simulink model "boost_rom_lpv_seed7"  (R2026a)
settings: Solver=ode1  StopTime=1.4  FixedStep=5e-07
PreLoadFcn:
  | mdlDir = fileparts(which('boost_rom_lpv_seed7'));
  | repoRoot = fileparts(mdlDir);
  | load(fullfile(repoRoot, 'model_data', 'boost_rom_lpv_seed7_data.mat'));
  | load(fullfile(repoRoot, 'model_data', 'comparison_duty_profile.mat'));
values from neighbouring files (symbols this model uses):
  node_state_ic = [Vout_init; iL_init]    [setup_comparison_profile.m]
undefined symbols (not defined in the file or in its folder): lut_delta_iL, lut_duty, net_lpv, node_u_mean, node_u_std, node_x_mean, node_x_std
libraries: dlconvfclib x3, dlactivationlib x2
settings Model: Creator=arkadiyturevskiy  LastModifiedBy=arkadiyturevskiy

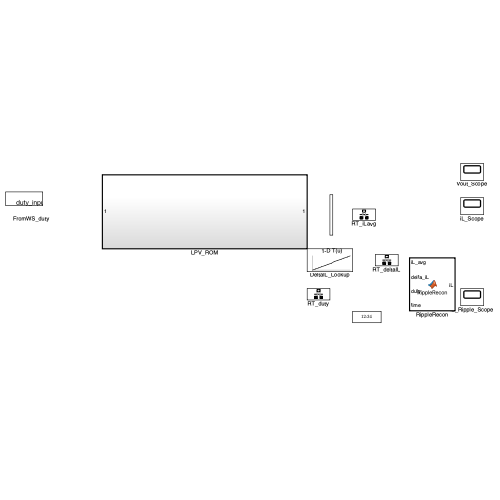
[thumbnail: Simulink's stored preview of the top-level diagram]
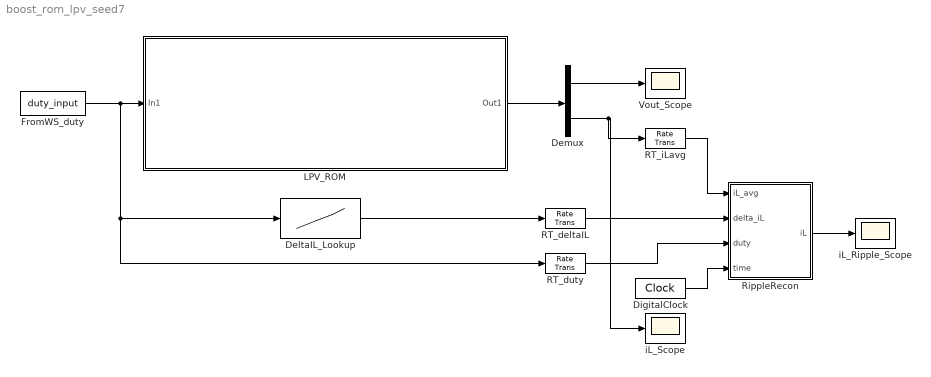
== system boost_rom_lpv_seed7 ==
  DeltaIL_Lookup : Lookup_n-D  NumberOfTableDimensions=1  BreakpointsForDimension1=lut_duty  Table=lut_delta_iL  ExtrapMethod=Clip  InternalRulePriority=Speed  RndMeth=Simplest
  Demux : Demux  Outputs=2
  DigitalClock : DigitalClock  SampleTime=5e-07
  FromWS_duty : FromWorkspace  VariableName=duty_input  OutputAfterFinalValue=Holding final value
  LPV_ROM : Subsystem  TreatAsAtomicUnit=on  SystemSampleTime=5e-06
  RT_deltaIL : RateTransition  OutPortSampleTime=5e-07
  RT_duty : RateTransition  OutPortSampleTime=5e-07
  RT_iLavg : RateTransition  OutPortSampleTime=5e-07
  RippleRecon : MATLAB Function  TreatAsAtomicUnit=on
  Vout_Scope : Scope
  iL_Ripple_Scope : Scope
  iL_Scope : Scope
  wires:
  RippleRecon/1(iL) -> iL_Ripple_Scope/1
  RT_iLavg/1 -> RippleRecon/1(iL_avg)
  RT_duty/1 -> RippleRecon/3(duty)
  RT_deltaIL/1 -> RippleRecon/2(delta_iL)
  Demux/2 -> RT_iLavg/1, iL_Scope/1
  FromWS_duty/1 -> DeltaIL_Lookup/1, RT_duty/1, LPV_ROM/1(In1)
  Demux/1 -> Vout_Scope/1
  DigitalClock/1 -> RippleRecon/4(time)
  DeltaIL_Lookup/1 -> RT_deltaIL/1
  LPV_ROM/1(Out1) -> Demux/1

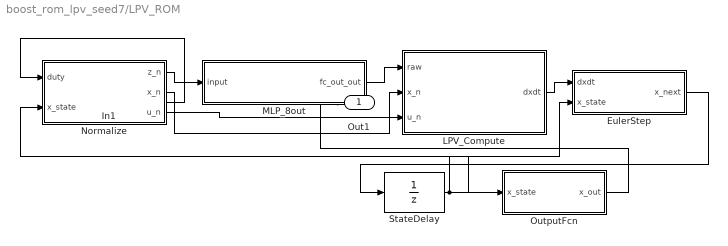
== system boost_rom_lpv_seed7/LPV_ROM ==
  In1 : Inport
  EulerStep : MATLAB Function  TreatAsAtomicUnit=on
  LPV_Compute : MATLAB Function  TreatAsAtomicUnit=on
  MLP_8out : Subsystem
  Normalize : MATLAB Function  TreatAsAtomicUnit=on
  OutputFcn : MATLAB Function  TreatAsAtomicUnit=on
  StateDelay : UnitDelay  InitialCondition=node_state_ic  SampleTime=5e-06
  Out1 : Outport
  wires:
  In1/1 -> Normalize/1(duty)
  StateDelay/1 -> Normalize/2(x_state), EulerStep/2(x_state), OutputFcn/1(x_state)
  Normalize/1(z_n) -> MLP_8out/1(input)
  MLP_8out/1(fc_out_out) -> LPV_Compute/1(raw)
  Normalize/2(x_n) -> LPV_Compute/2(x_n)
  Normalize/3(u_n) -> LPV_Compute/3(u_n)
  LPV_Compute/1(dxdt) -> EulerStep/1(dxdt)
  EulerStep/1(x_next) -> StateDelay/1
  OutputFcn/1(x_out) -> Out1/1

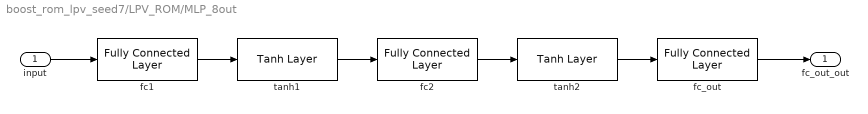
== system boost_rom_lpv_seed7/LPV_ROM/MLP_8out ==
  input : Inport  PortDimensions=[3]  SampleTime=5e-06
  fc1 : dlconvfclib/Fully Connected Layer  Layer=net_lpv.Layers(2)  OutMin=[]  OutMax=[]  WeightsDataTypeStr=Inherit: Inherit via back propagation  WeightsMin=[]  WeightsMax=[]  BiasDataTypeStr=Inherit: Inherit via back propagation  BiasMin=[]  BiasMax=[]  AccumMin=[]  AccumMax=[]  InternalRndMeth=Floor  InternalSaturateOnIntegerOverflow=off  SampleTime=5e-06
      settings: DataFormat=C
  fc2 : dlconvfclib/Fully Connected Layer  Layer=net_lpv.Layers(4)  OutMin=[]  OutMax=[]  WeightsDataTypeStr=Inherit: Inherit via back propagation  WeightsMin=[]  WeightsMax=[]  BiasDataTypeStr=Inherit: Inherit via back propagation  BiasMin=[]  BiasMax=[]  AccumMin=[]  AccumMax=[]  InternalRndMeth=Floor  InternalSaturateOnIntegerOverflow=off  SampleTime=5e-06
      settings: DataFormat=C
  fc_out : dlconvfclib/Fully Connected Layer  Layer=net_lpv.Layers(6)  OutMin=[]  OutMax=[]  WeightsDataTypeStr=Inherit: Inherit via back propagation  WeightsMin=[]  WeightsMax=[]  BiasDataTypeStr=Inherit: Inherit via back propagation  BiasMin=[]  BiasMax=[]  AccumMin=[]  AccumMax=[]  InternalRndMeth=Floor  InternalSaturateOnIntegerOverflow=off  SampleTime=5e-06
      settings: DataFormat=C
  tanh1 : dlactivationlib/Tanh Layer  ApproximationMethod=None  OutMin=[]  OutMax=[]  SampleTime=5e-06
  tanh2 : dlactivationlib/Tanh Layer  ApproximationMethod=None  OutMin=[]  OutMax=[]  SampleTime=5e-06
  fc_out_out : Outport
  wires:
  tanh2/1 -> fc_out/1
  tanh1/1 -> fc2/1
  fc1/1 -> tanh1/1
  input/1 -> fc1/1
  fc_out/1 -> fc_out_out/1
  fc2/1 -> tanh2/1

== matlab function boost_rom_lpv_seed7/LPV_ROM/LPV_Compute ==
  data: raw input; dxdt output; x_n input; u_n input; node_dxdt_scale parameter
function dxdt = LPV_Compute(raw, x_n, u_n, node_dxdt_scale)
%#codegen
% raw: 8-element vector [A(4), B(2), c(2)]
% x_n: 2-element normalized state
% u_n: scalar normalized input
A = reshape(raw(1:4), [2, 2]);
B = reshape(raw(5:6), [2, 1]);
c = raw(7:8);
dxdt_n = A * x_n + B * u_n + c;
dxdt = double(dxdt_n) .* node_dxdt_scale;

== matlab function boost_rom_lpv_seed7/LPV_ROM/Normalize ==
  data: duty input; z_n output; x_state input; x_n output; u_n output; node_x_mean parameter; node_x_std parameter; node_u_mean parameter; node_u_std parameter
function [z_n, x_n, u_n] = Normalize(duty, x_state, node_x_mean, node_x_std, node_u_mean, node_u_std)
%#codegen
x_n = (x_state - node_x_mean) ./ node_x_std;
u_n = (duty - node_u_mean) / node_u_std;
z_n = single([x_n; u_n]);

== matlab function boost_rom_lpv_seed7/LPV_ROM/EulerStep ==
  data: dxdt input; x_next output; x_state input
function x_next = EulerStep(dxdt, x_state)
%#codegen
Ts = 5.0000000000e-06;
x_next = x_state + Ts * dxdt;

== matlab function boost_rom_lpv_seed7/LPV_ROM/OutputFcn ==
  data: x_state input; x_out output
function x_out = OutputFcn(x_state)
%#codegen
x_out = x_state;

== matlab function boost_rom_lpv_seed7/RippleRecon ==
  data: iL_avg input; iL output; delta_iL input; duty input; time input
function iL = RippleRecon(iL_avg, delta_iL, duty, time)
%#codegen
Tsw = 5.0000000000e-06;
phase = mod(time, Tsw) / Tsw;
duty_c = max(0.01, min(0.99, duty));
if phase < duty_c
    iL = iL_avg - delta_iL/2 + delta_iL * (phase / duty_c);
else
    iL = iL_avg + delta_iL/2 - delta_iL * ((phase - duty_c) / (1 - duty_c + eps));
end
